simulink model "threepointfour"  (R2021a)
settings: Solver=VariableStepAuto  StartTime=0.0  StopTime=100  RelTol=1e-3
values from neighbouring files (symbols this model uses):
  k = 2    [Main.m]
undefined symbols (not defined in the file or in its folder): tao
settings Model: Creator=zd012  LastModifiedBy=zd012

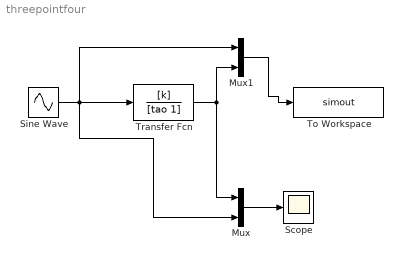
== system threepointfour ==
  Mux : Mux  Inputs=2
  Mux1 : Mux  Inputs=2
  Scope : Scope
  Sine Wave : Sin  SampleTime=0
  To Workspace : ToWorkspace  VariableName=simout  SaveFormat=Timeseries  SampleTime=-1
  Transfer Fcn : TransferFcn  Numerator=[k]  Denominator=[tao 1]
  wires:
  Sine Wave/1 -> Mux1/1, Mux/2, Transfer Fcn/1
  Transfer Fcn/1 -> Mux1/2, Mux/1
  Mux/1 -> Scope/1
  Mux1/1 -> To Workspace/1
